simulink model "DCM_estMc"  (R2020a)
settings: Solver=FixedStepAuto  StartTime=0.0  StopTime=2  FixedStep=1e-4  RelTol=1e-3
undefined symbols (not defined in the file): Idm, J, Ki_I, Ki_W, Kp_I, Kp_W, Kphi, Lu, Ru, Ubat
libraries: simulink x2
settings Model: Creator=Nguyen Tung  LastModifiedBy=Nguyen Tung

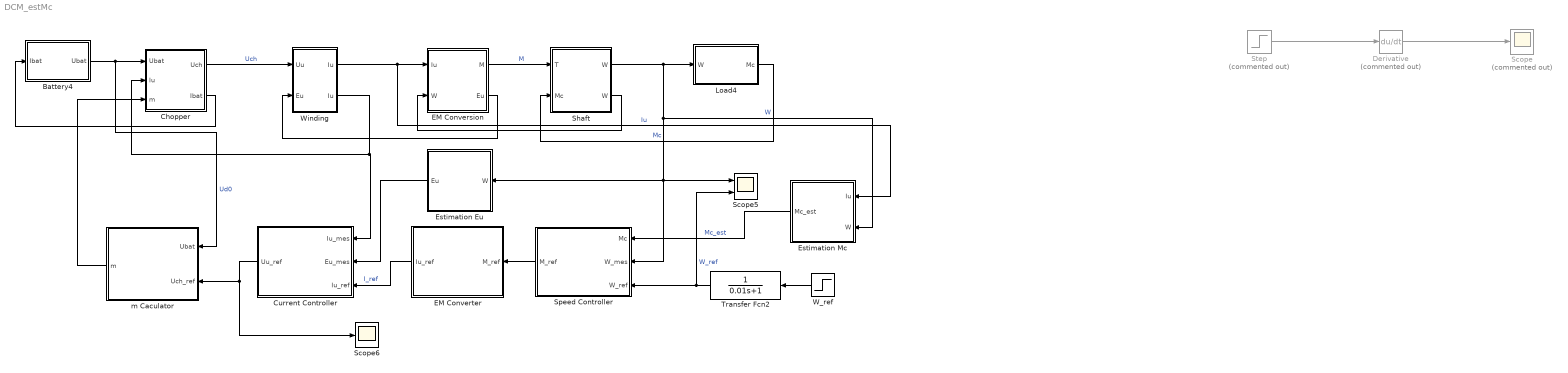
== system DCM_estMc ==
  Battery4 : Subsystem  AncestorBlock=simulink/REM/SE
      mask Display:
      | plot(0,0,100,100, 1.2*[50,57.68,60.77,63.08,64.97,66.58,68,69.26,70.4, 	71.42,72.36,78.28,80,78.28,72.36,71.42,70.4, 	69.26,68,66.58,64.97,63.08,60.77,57.68,50,42.32, 	39.23,36.92,35.03,33.42,32,30.74,29.6,28.58, 	27.64,21.72,20,21.72,27.64,28.58,29.6,30.74,32, 	33.42,35.03,36.92,39.23,42.32,50]-10, 1.2*[20,21,22,23,24,25,26,27,28,29,30,40,50,60,70,71,72, 	73,74,75,76,77,78,79,80,79,78,77,76,75,74,73,72, 	71,70,60,50,40,30,29,28,27,26,25,24,23,22,21,20]-10)
      | disp('ES')
  Chopper : Subsystem  AncestorBlock=simulink/REM/EC Elec  mask(Hacheur){}
      mask Display: plot(0,0,100,100,[10,10,90,90,10],[90,10,10,90,90])
  Current Controller : Subsystem  AncestorBlock=simulink/SMC/Asservissement Correcteur IP
      mask Display: plot(0,0,100,100, [10,30,90,70,10,90],[90,10,10,90,90,10])
  Derivative : Derivative  Commented=on  CoefficientInTFapproximation=1
  EM Conversion : Subsystem  AncestorBlock=simulink/REM/EC EM
      mask Display: plot(0,0,100,100, 1.4*[50,57.68,60.77,63.08,64.97,66.58,68,69.26,70.4, 	71.42,72.36,78.28,80,78.28,72.36,71.42,70.4, 	69.26,68,66.58,64.97,63.08,60.77,57.68,50,42.32, 	39.23,36.92,35.03,33.42,32,30.74,29.6,28.58, 	27.64,21.72,20,21.72,27.64,28.58,29.6,30.74,32, 	33.42,35.03,36.92,39.23,42.32,50]-20, 1.4*[20,21,22,23,24,25,26,27,28,29,30,40,50,60,70,71,72, 	73,74,75,76,77,78,79,80,79,78,77,76,75,74,73,72, 	71,70,60,50,40,30,29,28,27,26,25,24,23,22,21,20]-20)
  EM Converter : Subsystem  AncestorBlock=simulink/SMC/Inversion EC avec mesure
      mask Display: plot(0,0,100,100,[10,30,90,70,10],[90,10,10,90,90])
  Estimation Eu : Subsystem  AncestorBlock=simulink/REM/EC EM
      mask Display: plot(0,0,100,100, 1.4*[50,57.68,60.77,63.08,64.97,66.58,68,69.26,70.4, 	71.42,72.36,78.28,80,78.28,72.36,71.42,70.4, 	69.26,68,66.58,64.97,63.08,60.77,57.68,50,42.32, 	39.23,36.92,35.03,33.42,32,30.74,29.6,28.58, 	27.64,21.72,20,21.72,27.64,28.58,29.6,30.74,32, 	33.42,35.03,36.92,39.23,42.32,50]-20, 1.4*[20,21,22,23,24,25,26,27,28,29,30,40,50,60,70,71,72, 	73,74,75,76,77,78,79,80,79,78,77,76,75,74,73,72, 	71,70,60,50,40,30,29,28,27,26,25,24,23,22,21,20]-20)
  Estimation Mc : Subsystem  AncestorBlock=simulink/REM/EC EM
      mask Display: plot(0,0,100,100, 1.4*[50,57.68,60.77,63.08,64.97,66.58,68,69.26,70.4, 	71.42,72.36,78.28,80,78.28,72.36,71.42,70.4, 	69.26,68,66.58,64.97,63.08,60.77,57.68,50,42.32, 	39.23,36.92,35.03,33.42,32,30.74,29.6,28.58, 	27.64,21.72,20,21.72,27.64,28.58,29.6,30.74,32, 	33.42,35.03,36.92,39.23,42.32,50]-20, 1.4*[20,21,22,23,24,25,26,27,28,29,30,40,50,60,70,71,72, 	73,74,75,76,77,78,79,80,79,78,77,76,75,74,73,72, 	71,70,60,50,40,30,29,28,27,26,25,24,23,22,21,20]-20)
  Load4 : Subsystem  AncestorBlock=simulink/REM/SE
      mask Display:
      | plot(0,0,100,100, 1.2*[50,57.68,60.77,63.08,64.97,66.58,68,69.26,70.4, 	71.42,72.36,78.28,80,78.28,72.36,71.42,70.4, 	69.26,68,66.58,64.97,63.08,60.77,57.68,50,42.32, 	39.23,36.92,35.03,33.42,32,30.74,29.6,28.58, 	27.64,21.72,20,21.72,27.64,28.58,29.6,30.74,32, 	33.42,35.03,36.92,39.23,42.32,50]-10, 1.2*[20,21,22,23,24,25,26,27,28,29,30,40,50,60,70,71,72, 	73,74,75,76,77,78,79,80,79,78,77,76,75,74,73,72, 	71,70,60,50,40,30,29,28,27,26,25,24,23,22,21,20]-10)
      | disp('MS')
  Scope : Scope  Commented=on
  Scope5 : Scope  NumInputPorts=2
  Scope6 : Scope
  Shaft : Subsystem  AncestorBlock=simulink/REM/EA  mask(CM){}
      mask Display: plot(0,0,100,100,[10,10,90,90,10],[90,10,10,90,90], [10,90],[10,90])
  Speed Controller : Subsystem  AncestorBlock=simulink/SMC/Asservissement Correcteur IP
      mask Display: plot(0,0,100,100, [10,30,90,70,10,90],[90,10,10,90,90,10])
  Step : Step  Commented=on  SampleTime=0
  Transfer Fcn2 : TransferFcn  Denominator=[0.01 1]
  W_ref : Step  Time=0.5  After=50  SampleTime=0
  Winding : Subsystem  AncestorBlock=simulink/REM/EA  mask(CM){}
      mask Display: plot(0,0,100,100,[10,10,90,90,10],[90,10,10,90,90], [10,90],[10,90])
  m Caculator : Subsystem  AncestorBlock=simulink/SMC/Inversion EC avec mesure
      mask Display: plot(0,0,100,100,[10,30,90,70,10],[90,10,10,90,90])
  wires:
  Winding/2(Iu) -> Current Controller/1(Iu_mes), Chopper/2(Iu)
  Chopper/2(Ibat) -> Battery4/1(Ibat)
  Estimation Eu/1(Eu) -> Current Controller/2(Eu_mes)
  Transfer Fcn2/1 -> Speed Controller/3(W_ref), Scope5/2  "W_ref"
  Current Controller/1(Uu_ref) -> m Caculator/2(Uch_ref), Scope6/1
  EM Conversion/1(M) -> Shaft/1(T)  "M"
  EM Converter/1(Iu_ref) -> Current Controller/3(Iu_ref)  "I_ref"
  Speed Controller/1(M_ref) -> EM Converter/1(M_ref)
  m Caculator/1(m) -> Chopper/3(m)
  Load4/1(Mc) -> Shaft/2(Mc)  "Mc"
  Shaft/1(W) -> Load4/1(W), Estimation Mc/2(W), Scope5/1, Speed Controller/2(W_mes), Estimation Eu/1(W)  "W"
  W_ref/1 -> Transfer Fcn2/1
  Winding/1("Iu ") -> Estimation Mc/1(Iu), EM Conversion/1(Iu)  "Iu"
  Battery4/1(Ubat) -> m Caculator/1(Ubat), Chopper/1("Ubat ")  "Ud0"
  Chopper/1(Uch) -> Winding/1(Uu)  "Uch"
  EM Conversion/2(Eu) -> Winding/2(Eu)
  Shaft/2("W ") -> EM Conversion/2(W)
  Step/1 -> Derivative/1
  Derivative/1 -> Scope/1
  Estimation Mc/1(Mc_est) -> Speed Controller/1(Mc)  "Mc_est"

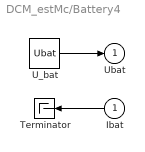
== system DCM_estMc/Battery4 ==
  Ibat : Inport
  Terminator : Terminator
  U_bat : Constant  Value=Ubat
  Ubat : Outport  InitialOutput=0  VectorParamsAs1DForOutWhenUnconnected=off
  wires:
  Ibat/1 -> Terminator/1
  U_bat/1 -> Ubat/1

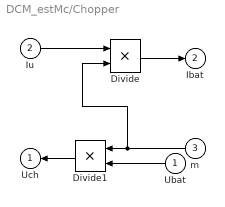
== system DCM_estMc/Chopper ==
  "Ubat " : Inport
  Iu : Inport  Port=2
  m : Inport  Port=3
  Divide : Product  Inputs=**
  Divide1 : Product  Inputs=**
  Uch : Outport  InitialOutput=0  VectorParamsAs1DForOutWhenUnconnected=off
  Ibat : Outport  Port=2  InitialOutput=0  VectorParamsAs1DForOutWhenUnconnected=off
  wires:
  m/1 -> Divide/2, Divide1/1
  Divide1/1 -> Uch/1
  "Ubat "/1 -> Divide1/2
  Divide/1 -> Ibat/1
  Iu/1 -> Divide/1

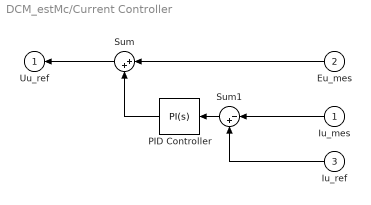
== system DCM_estMc/Current Controller ==
  Iu_mes : Inport
  Eu_mes : Inport  Port=2
  Iu_ref : Inport  Port=3
  PID Controller : simulink/Continuous/PID Controller  Controller=PI  Form=Parallel  TimeDomain=Continuous-time  UseExternalTs=off  SampleTime=-1  IntegratorMethod=Forward Euler  FilterMethod=Forward Euler  ControllerParametersSource=internal  P=Kp_I  I=Ki_I  D=0  UseFilter=on  N=100  TunerSelectOption=Transfer Function Based (PID Tuner App)  InitialConditionSource=internal  InitialConditionForIntegrator=0  InitialConditionForFilter=0  DifferentiatorICPrevScaledInput=0  ExternalReset=none  IgnoreLimit=on  TrackingMode=off  Kt=1  LimitOutput=off  UpperSaturationLimit=inf  LowerSaturationLimit=-inf  LinearizeAsGain=on  AntiWindupMode=none  Kb=1  POutMin=[]  POutMax=[]  IOutMin=[]  IOutMax=[]  DOutMin=[]  DOutMax=[]  NOutMin=[]  NOutMax=[]  SumOutMin=[]  SumOutMax=[]  SaturationOutMin=[]  SaturationOutMax=[]  PParamMin=[]  PParamMax=[]  IParamMin=[]  IParamMax=[]  DParamMin=[]  DParamMax=[]  NParamMin=[]  NParamMax=[]  KbParamMin=[]  KbParamMax=[]  KtParamMin=[]  KtParamMax=[]  KbOutMin=[]  KbOutMax=[]  KtOutMin=[]  KtOutMax=[]  IntegratorOutMin=[]  IntegratorOutMax=[]  FilterOutMin=[]  FilterOutMax=[]  SumI1OutMin=[]  SumI1OutMax=[]  SumI2OutMin=[]  SumI2OutMax=[]  SumI3OutMin=[]  SumI3OutMax=[]  SumI4OutMin=[]  SumI4OutMax=[]  SumDOutMin=[]  SumDOutMax=[]  DifferentiatorOutMin=[]  DifferentiatorOutMax=[]  FilterDiffOutCoefMin=[]  FilterDiffOutCoefMax=[]  ReciprocalOutMin=[]  ReciprocalOutMax=[]  SumDenOutMin=[]  SumDenOutMax=[]  SumNumOutMin=[]  SumNumOutMax=[]  DivideOutMin=[]  DivideOutMax=[]  UdiffTsProdOutMin=[]  UdiffTsProdOutMax=[]  NTsProdOutMin=[]  NTsProdOutMax=[]  UintegralTsProdOutMin=[]  UintegralTsProdOutMax=[]  UngainTsProdOutMin=[]  UngainTsProdOutMax=[]  IntegratorContinuousStateAttributes=''  IntegratorStateMustResolveToSignalObject=off  IntegratorRTWStateStorageClass=Auto  FilterContinuousStateAttributes=''  FilterStateMustResolveToSignalObject=off  FilterRTWStateStorageClass=Auto  ParallelPVariant=InternalParameters  IdealPVariant=Disabled  IVariant=InternalParameters  DVariant=Disabled  IntegratorVariant=Continuous  SatVariant=Disabled  AWVariant=Passthrough  PCopyVariant=Disabled  TRVariant=Disabled  FdbkBlocksVariant=Forward  IdealPFdbkVariant=Disabled  SatFdbkVariant=Disabled  DerivativeFilterVariant=Disabled  NVariant=Disabled  NCopyVariant=Disabled_SignalSpec  FilterICVariant=Disabled  IntegratorICVariant=InternalICs  ExternalResetVariant=Disabled  TRSumVariant=Passthrough  SumFdbkVariant=Disabled  SumVariant=Sum_PI  TsampFilterVariant=InternalTs  TsampNgainVariant=Passthrough  TsampIntegralVariant=Passthrough
  Sum : Sum  Inputs=|++
  Sum1 : Sum  Inputs=|-+
  Uu_ref : Outport  InitialOutput=0  VectorParamsAs1DForOutWhenUnconnected=off
  wires:
  Eu_mes/1 -> Sum/1
  Sum/1 -> Uu_ref/1
  Iu_mes/1 -> Sum1/1
  Sum1/1 -> PID Controller/1
  PID Controller/1 -> Sum/2
  Iu_ref/1 -> Sum1/2

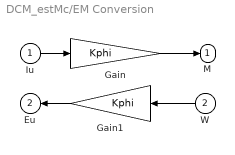
== system DCM_estMc/EM Conversion ==
  Iu : Inport
  W : Inport  Port=2
  Gain : Gain  Gain=Kphi
  Gain1 : Gain  Gain=Kphi
  M : Outport  InitialOutput=0  VectorParamsAs1DForOutWhenUnconnected=off
  Eu : Outport  Port=2  InitialOutput=0  VectorParamsAs1DForOutWhenUnconnected=off
  wires:
  Iu/1 -> Gain/1
  Gain/1 -> M/1
  W/1 -> Gain1/1
  Gain1/1 -> Eu/1

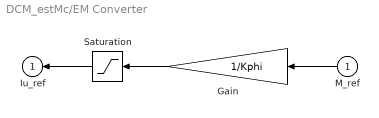
== system DCM_estMc/EM Converter ==
  M_ref : Inport
  Gain : Gain  Gain=1/Kphi
  Saturation : Saturate  UpperLimit=5*Idm  LowerLimit=-5*Idm
  Iu_ref : Outport  InitialOutput=0  VectorParamsAs1DForOutWhenUnconnected=off
  wires:
  M_ref/1 -> Gain/1
  Gain/1 -> Saturation/1
  Saturation/1 -> Iu_ref/1

== system DCM_estMc/Estimation Eu ==
  W : Inport
  Gain1 : Gain  Gain=Kphi
  Eu : Outport  InitialOutput=0  VectorParamsAs1DForOutWhenUnconnected=off
  wires:
  W/1 -> Gain1/1
  Gain1/1 -> Eu/1

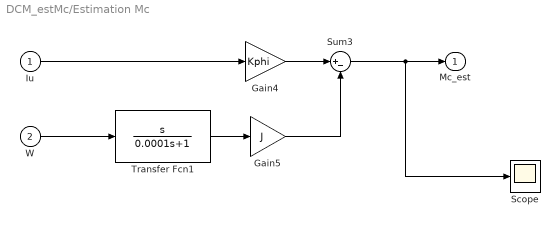
== system DCM_estMc/Estimation Mc ==
  Iu : Inport
  W : Inport  Port=2
  Gain4 : Gain  Gain=Kphi
  Gain5 : Gain  Gain=J
  Scope : Scope
  Sum3 : Sum  Inputs=|+-
  Transfer Fcn1 : TransferFcn  Numerator=[1 0]  Denominator=[0.0001 1]
  Mc_est : Outport  InitialOutput=0  VectorParamsAs1DForOutWhenUnconnected=off
  wires:
  Sum3/1 -> Scope/1, Mc_est/1
  Gain4/1 -> Sum3/1
  Transfer Fcn1/1 -> Gain5/1
  Iu/1 -> Gain4/1
  W/1 -> Transfer Fcn1/1
  Gain5/1 -> Sum3/2

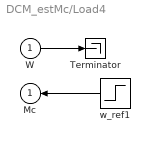
== system DCM_estMc/Load4 ==
  W : Inport
  Terminator : Terminator
  w_ref1 : Step  Time=1.5  After=30  SampleTime=0
  Mc : Outport  InitialOutput=0  VectorParamsAs1DForOutWhenUnconnected=off
  wires:
  W/1 -> Terminator/1
  w_ref1/1 -> Mc/1

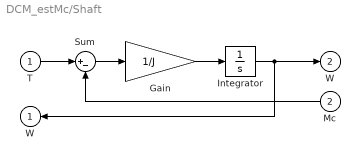
== system DCM_estMc/Shaft ==
  T : Inport
  Mc : Inport  Port=2
  Gain : Gain  Gain=1/J
  Integrator : Integrator  InitialCondition=0.001
  Sum : Sum  Inputs=|+-
  W : Outport  InitialOutput=0  VectorParamsAs1DForOutWhenUnconnected=off
  "W " : Outport  Port=2  InitialOutput=0  VectorParamsAs1DForOutWhenUnconnected=off
  wires:
  T/1 -> Sum/1
  Mc/1 -> Sum/2
  Sum/1 -> Gain/1
  Integrator/1 -> "W "/1, W/1
  Gain/1 -> Integrator/1

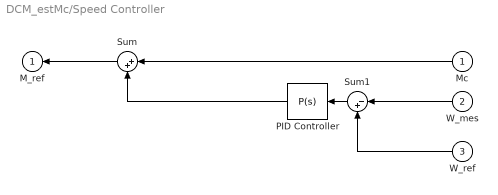
== system DCM_estMc/Speed Controller ==
  Mc : Inport
  W_mes : Inport  Port=2
  W_ref : Inport  Port=3
  PID Controller : simulink/Continuous/PID Controller  Controller=P  Form=Parallel  TimeDomain=Continuous-time  UseExternalTs=off  SampleTime=-1  IntegratorMethod=Forward Euler  FilterMethod=Forward Euler  ControllerParametersSource=internal  P=Kp_W  I=Ki_W  D=0  UseFilter=on  N=100  TunerSelectOption=Transfer Function Based (PID Tuner App)  InitialConditionSource=internal  InitialConditionForIntegrator=0  InitialConditionForFilter=0  DifferentiatorICPrevScaledInput=0  ExternalReset=none  TrackingMode=off  Kt=1  LimitOutput=off  UpperSaturationLimit=inf  LowerSaturationLimit=-inf  LinearizeAsGain=on  AntiWindupMode=none  Kb=1  POutMin=[]  POutMax=[]  IOutMin=[]  IOutMax=[]  DOutMin=[]  DOutMax=[]  NOutMin=[]  NOutMax=[]  SumOutMin=[]  SumOutMax=[]  SaturationOutMin=[]  SaturationOutMax=[]  PParamMin=[]  PParamMax=[]  IParamMin=[]  IParamMax=[]  DParamMin=[]  DParamMax=[]  NParamMin=[]  NParamMax=[]  KbParamMin=[]  KbParamMax=[]  KtParamMin=[]  KtParamMax=[]  KbOutMin=[]  KbOutMax=[]  KtOutMin=[]  KtOutMax=[]  IntegratorOutMin=[]  IntegratorOutMax=[]  FilterOutMin=[]  FilterOutMax=[]  SumI1OutMin=[]  SumI1OutMax=[]  SumI2OutMin=[]  SumI2OutMax=[]  SumI3OutMin=[]  SumI3OutMax=[]  SumI4OutMin=[]  SumI4OutMax=[]  SumDOutMin=[]  SumDOutMax=[]  DifferentiatorOutMin=[]  DifferentiatorOutMax=[]  FilterDiffOutCoefMin=[]  FilterDiffOutCoefMax=[]  ReciprocalOutMin=[]  ReciprocalOutMax=[]  SumDenOutMin=[]  SumDenOutMax=[]  SumNumOutMin=[]  SumNumOutMax=[]  DivideOutMin=[]  DivideOutMax=[]  UdiffTsProdOutMin=[]  UdiffTsProdOutMax=[]  NTsProdOutMin=[]  NTsProdOutMax=[]  UintegralTsProdOutMin=[]  UintegralTsProdOutMax=[]  UngainTsProdOutMin=[]  UngainTsProdOutMax=[]  IntegratorContinuousStateAttributes=''  IntegratorStateMustResolveToSignalObject=off  IntegratorRTWStateStorageClass=Auto  FilterContinuousStateAttributes=''  FilterStateMustResolveToSignalObject=off  FilterRTWStateStorageClass=Auto  ParallelPVariant=InternalParameters  IdealPVariant=Disabled  IVariant=Disabled  DVariant=Disabled  IntegratorVariant=Disabled  SatVariant=Disabled  AWVariant=Disabled  PCopyVariant=Disabled  TRVariant=Disabled  FdbkBlocksVariant=Forward  IdealPFdbkVariant=Disabled  SatFdbkVariant=Disabled  DerivativeFilterVariant=Disabled  NVariant=Disabled  NCopyVariant=Disabled_SignalSpec  FilterICVariant=Disabled  IntegratorICVariant=Disabled  ExternalResetVariant=Disabled  TRSumVariant=Passthrough  SumFdbkVariant=Disabled  SumVariant=Passthrough_P  TsampFilterVariant=InternalTs  TsampNgainVariant=Passthrough  TsampIntegralVariant=Disabled_SignalSpec
  Sum : Sum  Inputs=|++
  Sum1 : Sum  Inputs=|-+
  M_ref : Outport  InitialOutput=0  VectorParamsAs1DForOutWhenUnconnected=off
  wires:
  Sum/1 -> M_ref/1
  W_mes/1 -> Sum1/1
  W_ref/1 -> Sum1/2
  Sum1/1 -> PID Controller/1
  PID Controller/1 -> Sum/2
  Mc/1 -> Sum/1

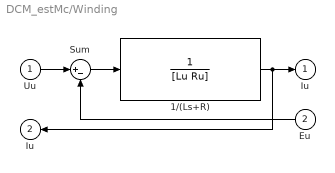
== system DCM_estMc/Winding ==
  Uu : Inport
  Eu : Inport  Port=2
  1/(Ls+R) : TransferFcn  Denominator=[Lu Ru]
  Sum : Sum  Inputs=|+-
  "Iu " : Outport  InitialOutput=0  VectorParamsAs1DForOutWhenUnconnected=off
  Iu : Outport  Port=2  InitialOutput=0  VectorParamsAs1DForOutWhenUnconnected=off
  wires:
  Uu/1 -> Sum/1
  Eu/1 -> Sum/2
  Sum/1 -> 1/(Ls+R)/1
  1/(Ls+R)/1 -> Iu/1, "Iu "/1

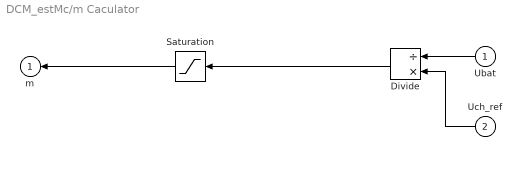
== system DCM_estMc/m Caculator ==
  Ubat : Inport
  Uch_ref : Inport  Port=2
  Divide : Product  Inputs=/*
  Saturation : Saturate  UpperLimit=1  LowerLimit=-1
  m : Outport  InitialOutput=0  VectorParamsAs1DForOutWhenUnconnected=off
  wires:
  Divide/1 -> Saturation/1
  Ubat/1 -> Divide/1
  Uch_ref/1 -> Divide/2
  Saturation/1 -> m/1
